simulink model "gm_uz_mpc_cost_and_optim_state_machine"  (R2021a)
settings: Solver=FixedStepAuto  StartTime=0.0  StopTime=10000*t_ADC  RelTol=1e-3
undefined symbols (not defined in the file or in its folder): A, f, IB, id_ref, iq_ref, ix_ref, iy_ref, lambda_d, lambda_q, lambda_u, lambda_x, lambda_y, Ld_over_LB, Lq_over_LB, n_rpm, omega_m, omegaB, p, psi_pm_over_psiB, Rs_over_ZB, t_ADC, t_clock, Ts_times_ZB_over_Ld, Ts_times_ZB_over_Lq, Ts_times_ZB_over_Lx, Ts_times_ZB_over_Ly, v_dc, VB
libraries: hdlmdlgenlib x73, nesl_utility x38, fl_lib x30, ee_lib x14, simulink x10, hdlsllib x2
(part 3 of 3)

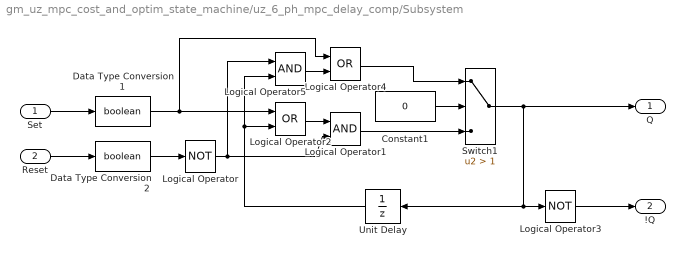
== system gm_uz_mpc_cost_and_optim_state_machine/uz_6_ph_mpc_delay_comp/Subsystem ==
  Set : Inport
  Reset : Inport  Port=2
  Constant1 : Constant  Value=0  OutDataTypeStr=uint32  SampleTime=-1
  Data Type Conversion1 : DataTypeConversion  OutDataTypeStr=boolean
  Data Type Conversion2 : DataTypeConversion  OutDataTypeStr=boolean
  Logical Operator : Logic  Operator=NOT  AllPortsSameDT=off  OutDataTypeStr=boolean
  Logical Operator1 : Logic  AllPortsSameDT=off  OutDataTypeStr=boolean
  Logical Operator2 : Logic  Operator=OR  AllPortsSameDT=off  OutDataTypeStr=boolean
  Logical Operator3 : Logic  Operator=NOT  AllPortsSameDT=off  OutDataTypeStr=boolean
  Logical Operator4 : Logic  Operator=OR  AllPortsSameDT=off  OutDataTypeStr=boolean
  Logical Operator5 : Logic  AllPortsSameDT=off  OutDataTypeStr=boolean
  Switch1 : Switch  Criteria=u2 > Threshold  Threshold=1
  Unit Delay : UnitDelay  InitialCondition=1  SampleTime=t_clock  HasFrameUpgradeWarning=on
  Q : Outport  VectorParamsAs1DForOutWhenUnconnected=off
  !Q : Outport  Port=2  VectorParamsAs1DForOutWhenUnconnected=off
  wires:
  Data Type Conversion2/1 -> Logical Operator/1
  Logical Operator1/1 -> Switch1/3
  Logical Operator5/1 -> Logical Operator4/2
  Unit Delay/1 -> Logical Operator5/2, Logical Operator2/2
  Logical Operator2/1 -> Logical Operator1/1
  Set/1 -> Data Type Conversion1/1
  Logical Operator3/1 -> !Q/1
  Switch1/1 -> Logical Operator3/1, Unit Delay/1, Q/1
  Data Type Conversion1/1 -> Logical Operator4/1, Logical Operator2/1
  Logical Operator4/1 -> Switch1/1
  Constant1/1 -> Switch1/2
  Reset/1 -> Data Type Conversion2/1
  Logical Operator/1 -> Logical Operator5/1, Logical Operator1/2

== system gm_uz_mpc_cost_and_optim_state_machine/uz_6ph_mpc_costs_and_optimization/FiniteControlSetSwitchingTable ==
  FiniteControlSetSwitchingTable : MATLAB Function  TreatAsAtomicUnit=on
  G : Outport  SampleTime=1e-08
  wires:
  FiniteControlSetSwitchingTable/1(G) -> G/1

== system gm_uz_mpc_cost_and_optim_state_machine/uz_6ph_mpc_costs_and_optimization/MATLAB Function ==
  in : Inport  OutDataTypeStr=boolean  PortDimensions=[64,12]  SampleTime=1e-08
  index : Inport  Port=2  OutDataTypeStr=uint8  PortDimensions=1  SampleTime=1e-08
  last_optim_index : Inport  Port=3  OutDataTypeStr=uint32  PortDimensions=1  SampleTime=1e-08
  MATLAB Function : MATLAB Function  TreatAsAtomicUnit=on
  G_next : Outport  SampleTime=1e-08  VectorParamsAs1DForOutWhenUnconnected=off
  G_prev : Outport  Port=2  SampleTime=1e-08
  wires:
  in/1 -> MATLAB Function/1(in)
  index/1 -> MATLAB Function/2(index)
  last_optim_index/1 -> MATLAB Function/3(last_optim_index)
  MATLAB Function/1(G_next) -> G_next/1
  MATLAB Function/2(G_prev) -> G_prev/1

== system gm_uz_mpc_cost_and_optim_state_machine/uz_6ph_mpc_costs_and_optimization/iterativesearch ==
  index : Inport  OutDataTypeStr=uint8  PortDimensions=1  SampleTime=1e-08
  cost : Inport  Port=2  OutDataTypeStr=fixdt(0, 27, 24)  PortDimensions=1  SampleTime=1e-08
  iterativesearch : MATLAB Function  TreatAsAtomicUnit=on
  iterativesearch_term1 : Terminator
  opt_idx : Outport  SampleTime=1e-08  VectorParamsAs1DForOutWhenUnconnected=off
  wires:
  index/1 -> iterativesearch/1(index)
  cost/1 -> iterativesearch/2(cost)
  iterativesearch/1(opt_idx) -> opt_idx/1
  iterativesearch/2(min_costs) -> iterativesearch_term1/1

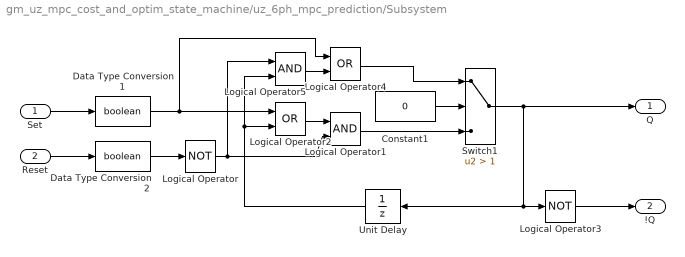
== system gm_uz_mpc_cost_and_optim_state_machine/uz_6ph_mpc_prediction/Subsystem ==
  Set : Inport
  Reset : Inport  Port=2
  Constant1 : Constant  Value=0  OutDataTypeStr=uint32  SampleTime=-1
  Data Type Conversion1 : DataTypeConversion  OutDataTypeStr=boolean
  Data Type Conversion2 : DataTypeConversion  OutDataTypeStr=boolean
  Logical Operator : Logic  Operator=NOT  AllPortsSameDT=off  OutDataTypeStr=boolean
  Logical Operator1 : Logic  AllPortsSameDT=off  OutDataTypeStr=boolean
  Logical Operator2 : Logic  Operator=OR  AllPortsSameDT=off  OutDataTypeStr=boolean
  Logical Operator3 : Logic  Operator=NOT  AllPortsSameDT=off  OutDataTypeStr=boolean
  Logical Operator4 : Logic  Operator=OR  AllPortsSameDT=off  OutDataTypeStr=boolean
  Logical Operator5 : Logic  AllPortsSameDT=off  OutDataTypeStr=boolean
  Switch1 : Switch  Criteria=u2 > Threshold  Threshold=1
  Unit Delay : UnitDelay  SampleTime=t_clock  HasFrameUpgradeWarning=on
  Q : Outport  VectorParamsAs1DForOutWhenUnconnected=off
  !Q : Outport  Port=2  VectorParamsAs1DForOutWhenUnconnected=off
  wires:
  Data Type Conversion2/1 -> Logical Operator/1
  Logical Operator1/1 -> Switch1/3
  Logical Operator5/1 -> Logical Operator4/2
  Unit Delay/1 -> Logical Operator5/2, Logical Operator2/2
  Logical Operator2/1 -> Logical Operator1/1
  Set/1 -> Data Type Conversion1/1
  Logical Operator3/1 -> !Q/1
  Switch1/1 -> Logical Operator3/1, Unit Delay/1, Q/1
  Data Type Conversion1/1 -> Logical Operator4/1, Logical Operator2/1
  Logical Operator4/1 -> Switch1/1
  Constant1/1 -> Switch1/2
  Reset/1 -> Data Type Conversion2/1
  Logical Operator/1 -> Logical Operator5/1, Logical Operator1/2

== system gm_uz_mpc_cost_and_optim_state_machine/uz_6ph_mpc_pu_voltages_vsd/Subsystem ==
  Set : Inport
  Reset : Inport  Port=2
  Constant1 : Constant  Value=0  OutDataTypeStr=uint32  SampleTime=-1
  Data Type Conversion1 : DataTypeConversion  OutDataTypeStr=boolean
  Data Type Conversion2 : DataTypeConversion  OutDataTypeStr=boolean
  Logical Operator : Logic  Operator=NOT  AllPortsSameDT=off  OutDataTypeStr=boolean
  Logical Operator1 : Logic  AllPortsSameDT=off  OutDataTypeStr=boolean
  Logical Operator2 : Logic  Operator=OR  AllPortsSameDT=off  OutDataTypeStr=boolean
  Logical Operator3 : Logic  Operator=NOT  AllPortsSameDT=off  OutDataTypeStr=boolean
  Logical Operator4 : Logic  Operator=OR  AllPortsSameDT=off  OutDataTypeStr=boolean
  Logical Operator5 : Logic  AllPortsSameDT=off  OutDataTypeStr=boolean
  Switch1 : Switch  Criteria=u2 > Threshold  Threshold=1
  Unit Delay : UnitDelay  SampleTime=t_clock  HasFrameUpgradeWarning=on
  Q : Outport  VectorParamsAs1DForOutWhenUnconnected=off
  !Q : Outport  Port=2  VectorParamsAs1DForOutWhenUnconnected=off
  wires:
  Data Type Conversion2/1 -> Logical Operator/1
  Logical Operator1/1 -> Switch1/3
  Logical Operator5/1 -> Logical Operator4/2
  Unit Delay/1 -> Logical Operator5/2, Logical Operator2/2
  Logical Operator2/1 -> Logical Operator1/1
  Set/1 -> Data Type Conversion1/1
  Logical Operator3/1 -> !Q/1
  Switch1/1 -> Logical Operator3/1, Unit Delay/1, Q/1
  Data Type Conversion1/1 -> Logical Operator4/1, Logical Operator2/1
  Logical Operator4/1 -> Switch1/1
  Constant1/1 -> Switch1/2
  Reset/1 -> Data Type Conversion2/1
  Logical Operator/1 -> Logical Operator5/1, Logical Operator1/2

== matlab function gm_uz_mpc_cost_and_optim_state_machine/uz_6ph_mpc_pu_voltages_vsd/finite_control_set ==
  settings: fimath=fimath('RoundingMethod', 'Floor','OverflowAction', 'Wrap','ProductMode', 'FullPrecision', 'SumMode', 'FullPrecision')
  data: v_DC_pu input; sin_angle input; pu_ud output; pu_uq output; pu_ux output; pu_uy output; cos_angle input; index input
function [pu_ud,pu_uq,pu_ux,pu_uy] = voltage_space_vectors(v_DC_pu, sin_angle, cos_angle, index)

fm = fimath();
v_DC_pu = fi(v_DC_pu,1,18,15,fm);
sin_angle = fi(sin_angle,1,18,16,fm);
cos_angle = fi(cos_angle,1,18,16,fm);

% u_d-voltages lookup factors alpha/beta
vd_pu = fi([0.000000,  0.000000;
0.333333,  -0.000000;
-0.166667,  0.288675;
0.166667,  0.288675;
-0.166667,  -0.288675;
0.166667,  -0.288675;
-0.333333,  0.000000;
0.000000,  0.000000;
0.288675,  0.166667;
0.622008,  0.166667;
0.122008,  0.455342;
0.455342,  0.455342;
0.122008,  -0.122008;
0.455342,  -0.122008;
-0.044658,  0.166667;
0.288675,  0.166667;
-0.288675,  0.166667;
0.044658,  0.166667;
-0.455342,  0.455342;
-0.122008,  0.455342;
-0.455342,  -0.122008;
-0.122008,  -0.122008;
-0.622008,  0.166667;
-0.288675,  0.166667;
0.000000,  0.333333;
0.333333,  0.333333;
-0.166667,  0.622008;
0.166667,  0.622008;
-0.166667,  0.044658;
0.166667,  0.044658;
-0.333333,  0.333333;
0.000000,  0.333333;
-0.000000,  -0.333333;
0.333333,  -0.333333;
-0.166667,  -0.044658;
0.166667,  -0.044658;
-0.166667,  -0.622008;
0.166667,  -0.622008;
-0.333333,  -0.333333;
-0.000000,  -0.333333;
0.288675,  -0.166667;
0.622008,  -0.166667;
0.122008,  0.122008;
0.455342,  0.122008;
0.122008,  -0.455342;
0.455342,  -0.455342;
-0.044658,  -0.166667;
0.288675,  -0.166667;
-0.288675,  -0.166667;
0.044658,  -0.166667;
-0.455342,  0.122008;
-0.122008,  0.122008;
-0.455342,  -0.455342;
-0.122008,  -0.455342;
-0.622008,  -0.166667;
-0.288675,  -0.166667;
0.000000,  0.000000;
0.333333,  -0.000000;
-0.166667,  0.288675;
0.166667,  0.288675;
-0.166667,  -0.288675;
0.166667,  -0.288675;
-0.333333,  0.000000;
0.000000,  0.000000],1,18,15);

% u_q-voltages lookup factors alpha/beta
vq_pu = fi([0.000000, 0.000000;
0.333333, -0.000000;
-0.166667, 0.288675;
0.166667, 0.288675;
-0.166667, -0.288675;
0.166667, -0.288675;
-0.333333, 0.000000;
0.000000, 0.000000;
0.288675, 0.166667;
0.622008, 0.166667;
0.122008, 0.455342;
0.455342, 0.455342;
0.122008, -0.122008;
0.455342, -0.122008;
-0.044658, 0.166667;
0.288675, 0.166667;
-0.288675, 0.166667;
0.044658, 0.166667;
-0.455342, 0.455342;
-0.122008, 0.455342;
-0.455342, -0.122008;
-0.122008, -0.122008;
-0.622008, 0.166667;
-0.288675, 0.166667;
0.000000, 0.333333;
0.333333, 0.333333;
-0.166667, 0.622008;
0.166667, 0.622008;
-0.166667, 0.044658;
0.166667, 0.044658;
-0.333333, 0.333333;
0.000000, 0.333333;
-0.000000, -0.333333;
0.333333, -0.333333;
-0.166667, -0.044658;
0.166667, -0.044658;
-0.166667, -0.622008;
0.166667, -0.622008;
-0.333333, -0.333333;
-0.000000, -0.333333;
0.288675, -0.166667;
0.622008, -0.166667;
0.122008, 0.122008;
0.455342, 0.122008;
0.122008, -0.455342;
0.455342, -0.455342;
-0.044658, -0.166667;
0.288675, -0.166667;
-0.288675, -0.166667;
0.044658, -0.166667;
-0.455342, 0.122008;
-0.122008, 0.122008;
-0.455342, -0.455342;
-0.122008, -0.455342;
-0.622008, -0.166667;
-0.288675, -0.166667;
0.000000, 0.000000;
0.333333, -0.000000;
-0.166667, 0.288675;
0.166667, 0.288675;
-0.166667, -0.288675;
0.166667, -0.288675;
-0.333333, 0.000000;
0.000000, 0.000000],1,18,15);
     
% u_x-voltages
vx_pu = fi([0.000000;
0.333333;
-0.166667;
0.166667;
-0.166667;
0.166667;
-0.333333;
0.000000;
-0.288675;
0.044658;
-0.455342;
-0.122008;
-0.455342;
-0.122008;
-0.622008;
-0.288675;
0.288675;
0.622008;
0.122008;
0.455342;
0.122008;
0.455342;
-0.044658;
0.288675;
0.000000;
0.333333;
-0.166667;
0.166667;
-0.166667;
0.166667;
-0.333333;
0.000000;
-0.000000;
0.333333;
-0.166667;
0.166667;
-0.166667;
0.166667;
-0.333333;
-0.000000;
-0.288675;
0.044658;
-0.455342;
-0.122008;
-0.455342;
-0.122008;
-0.622008;
-0.288675;
0.288675;
0.622008;
0.122008;
0.455342;
0.122008;
0.455342;
-0.044658;
0.288675;
0.000000;
0.333333;
-0.166667;
0.166667;
-0.166667;
0.166667;
-0.333333;
0.000000],1,18,15);

% u_y-voltages
vy_pu = fi([0.000000;
-0.000000;
-0.288675;
-0.288675;
0.288675;
0.288675;
0.000000;
0.000000;
0.166667;
0.166667;
-0.122008;
-0.122008;
0.455342;
0.455342;
0.166667;
0.166667;
0.166667;
0.166667;
-0.122008;
-0.122008;
0.455342;
0.455342;
0.166667;
0.166667;
0.333333;
0.333333;
0.044658;
0.044658;
0.622008;
0.622008;
0.333333;
0.333333;
-0.333333;
-0.333333;
-0.622008;
-0.622008;
-0.044658;
-0.044658;
-0.333333;
-0.333333;
-0.166667;
-0.166667;
-0.455342;
-0.455342;
0.122008;
0.122008;
-0.166667;
-0.166667;
-0.166667;
-0.166667;
-0.455342;
-0.455342;
0.122008;
0.122008;
-0.166667;
-0.166667;
0.000000;
-0.000000;
-0.288675;
-0.288675;
0.288675;
0.288675;
0.000000;
0.000000],1,18,15);

pu_ud = fi(v_DC_pu * (vd_pu(index,1) * cos_angle + vd_pu(index,2) * sin_angle),1,27,24);
pu_uq = fi(v_DC_pu * (vq_pu(index,1) * -sin_angle + vq_pu(index,2) * cos_angle),1,27,24);
pu_ux = fi(v_DC_pu * vx_pu(index),1,27,24);
pu_uy = fi(v_DC_pu * vy_pu(index),1,27,24);

== matlab function gm_uz_mpc_cost_and_optim_state_machine/uz_vsd_6ph_30deg/VSD_6ph_30deg ==
  settings: fimath=fimath('RoundingMethod', 'Floor','OverflowAction', 'Wrap','ProductMode', 'FullPrecision', 'SumMode', 'FullPrecision')
  data: a1 input; alpha output; b1 input; c1 input; a2 input; b2 input; c2 input; beta output; x1 output; y1 output; z1 output; z2 output
function [alpha,beta,x1,y1,z1,z2] = fcn(a1,b1,c1,a2,b2,c2)


A = [fi(0,1,18,11) fi(0,1,18,11) fi(0,1,18,11) fi(0,1,18,11) fi(0,1,18,11) fi(0,1,18,11)]';

A =    2/6*[1    -0.5        -0.5        sqrt(3)/2   -sqrt(3)/2  0 ;
           0    sqrt(3)/2   -sqrt(3)/2  0.5         0.5         -1;
           1    -0.5        -0.5        -sqrt(3)/2  sqrt(3)/2   0 ;
           0    -sqrt(3)/2  sqrt(3)/2   0.5         0.5         -1;
           0.5   0.5          0.5          0           0           0 ;
           0    0           0           0.5          0.5          0.5] * [a1 b1 c1 a2 b2 c2]';

alpha = fi(A(1),1,18,11);
beta = fi(A(2),1,18,11);
x1 = fi(A(3),1,18,11);
y1 = fi(A(4),1,18,11);
z1 = fi(A(5),1,18,11);
z2 = fi(A(6),1,18,11);

== matlab function gm_uz_mpc_cost_and_optim_state_machine/uz_6ph_mpc_costs_and_optimization/MATLAB Function/MATLAB Function ==
  settings: fimath=fimath('RoundingMethod', 'Floor','OverflowAction', 'Wrap','ProductMode', 'FullPrecision', 'SumMode', 'FullPrecision')
  data: in input; G_next output; index input; last_optim_index input; G_prev output
function [G_next,G_prev] = get_switch_positions(in,index,last_optim_index)
%#codegen
G_next = in(index,[1 3 5 7 9 11]);
G_prev = in(last_optim_index,[1 3 5 7 9 11]);

== matlab function gm_uz_mpc_cost_and_optim_state_machine/uz_6ph_mpc_costs_and_optimization/iterativesearch/iterativesearch ==
  data: index input; opt_idx output; cost input; min_costs output
function [opt_idx,min_costs] = fcn(index, cost)
%#codegen

persistent cost_old
if isempty(cost_old)
    cost_old = fi(4.98,0,27,24);
end

persistent index_old
if isempty(index_old)
    index_old = uint8(1);
end

persistent opt_idx_old
if isempty(opt_idx_old)
    opt_idx_old = uint8(1);
end


if (index < 63)       
       
if (index ~= index_old)
   if (cost <= cost_old)
       opt_idx_old = index; 
       cost_old = cost;
   else
    
    
   end
   index_old = index;
end

else
       cost_old = fi(4.98,0,27,24);
end

min_costs = cost_old;
opt_idx = opt_idx_old;

== matlab function gm_uz_mpc_cost_and_optim_state_machine/uz_6ph_mpc_costs_and_optimization/FiniteControlSetSwitchingTable/FiniteControlSetSwitchingTable ==
  settings: fimath=fimath('RoundingMethod', 'Floor','OverflowAction', 'Wrap','ProductMode', 'FullPrecision', 'SumMode', 'FullPrecision')
  data: G output
function G  = switchingTable

% -------------------------------------------------------------------
%  Generated by MATLAB on 14-Oct-2020 14:52:37
%  MATLAB version: 9.4.0.813654 (R2018a)
% -------------------------------------------------------------------
                                         

s1_v = boolean([0; 1; 0; 1; 0; 1; 0; 1; 0; 1; 0; 1; 0; 1; 0; 1; 0; 1; 0; 1; 0; ...
        1; 0; 1; 0; 1; 0; 1; 0; 1; 0; 1; 0; 1; 0; 1; 0; 1; 0; 1; 0; 1; ...
        0; 1; 0; 1; 0; 1; 0; 1; 0; 1; 0; 1; 0; 1; 0; 1; 0; 1; 0; 1; 0; ...
        1]);


s2_v = boolean([1; 0; 1; 0; 1; 0; 1; 0; 1; 0; 1; 0; 1; 0; 1; 0; 1; 0; 1; 0; 1; ...
        0; 1; 0; 1; 0; 1; 0; 1; 0; 1; 0; 1; 0; 1; 0; 1; 0; 1; 0; 1; 0; ...
        1; 0; 1; 0; 1; 0; 1; 0; 1; 0; 1; 0; 1; 0; 1; 0; 1; 0; 1; 0; 1; ...
        0]);


s3_v = boolean([0; 0; 1; 1; 0; 0; 1; 1; 0; 0; 1; 1; 0; 0; 1; 1; 0; 0; 1; 1; 0; ...
        0; 1; 1; 0; 0; 1; 1; 0; 0; 1; 1; 0; 0; 1; 1; 0; 0; 1; 1; 0; 0; ...
        1; 1; 0; 0; 1; 1; 0; 0; 1; 1; 0; 0; 1; 1; 0; 0; 1; 1; 0; 0; 1; ...
        1]);


s4_v = boolean([1; 1; 0; 0; 1; 1; 0; 0; 1; 1; 0; 0; 1; 1; 0; 0; 1; 1; 0; 0; 1; ...
        1; 0; 0; 1; 1; 0; 0; 1; 1; 0; 0; 1; 1; 0; 0; 1; 1; 0; 0; 1; 1; ...
        0; 0; 1; 1; 0; 0; 1; 1; 0; 0; 1; 1; 0; 0; 1; 1; 0; 0; 1; 1; 0; ...
        0]);


s5_v = boolean([0; 0; 0; 0; 1; 1; 1; 1; 0; 0; 0; 0; 1; 1; 1; 1; 0; 0; 0; 0; 1; ...
        1; 1; 1; 0; 0; 0; 0; 1; 1; 1; 1; 0; 0; 0; 0; 1; 1; 1; 1; 0; 0; ...
        0; 0; 1; 1; 1; 1; 0; 0; 0; 0; 1; 1; 1; 1; 0; 0; 0; 0; 1; 1; 1; ...
        1]);


s6_v = boolean([1; 1; 1; 1; 0; 0; 0; 0; 1; 1; 1; 1; 0; 0; 0; 0; 1; 1; 1; 1; 0; ...
        0; 0; 0; 1; 1; 1; 1; 0; 0; 0; 0; 1; 1; 1; 1; 0; 0; 0; 0; 1; 1; ...
        1; 1; 0; 0; 0; 0; 1; 1; 1; 1; 0; 0; 0; 0; 1; 1; 1; 1; 0; 0; 0; ...
        0]);


s7_v = boolean([0; 0; 0; 0; 0; 0; 0; 0; 1; 1; 1; 1; 1; 1; 1; 1; 0; 0; 0; 0; 0; ...
        0; 0; 0; 1; 1; 1; 1; 1; 1; 1; 1; 0; 0; 0; 0; 0; 0; 0; 0; 1; 1; ...
        1; 1; 1; 1; 1; 1; 0; 0; 0; 0; 0; 0; 0; 0; 1; 1; 1; 1; 1; 1; 1; ...
        1]);


s8_v = boolean([1; 1; 1; 1; 1; 1; 1; 1; 0; 0; 0; 0; 0; 0; 0; 0; 1; 1; 1; 1; 1; ...
        1; 1; 1; 0; 0; 0; 0; 0; 0; 0; 0; 1; 1; 1; 1; 1; 1; 1; 1; 0; 0; ...
        0; 0; 0; 0; 0; 0; 1; 1; 1; 1; 1; 1; 1; 1; 0; 0; 0; 0; 0; 0; 0; ...
        0]);


s9_v = boolean([0; 0; 0; 0; 0; 0; 0; 0; 0; 0; 0; 0; 0; 0; 0; 0; 1; 1; 1; 1; 1; ...
        1; 1; 1; 1; 1; 1; 1; 1; 1; 1; 1; 0; 0; 0; 0; 0; 0; 0; 0; 0; 0; ...
        0; 0; 0; 0; 0; 0; 1; 1; 1; 1; 1; 1; 1; 1; 1; 1; 1; 1; 1; 1; 1; ...
        1]);


s10_v = boolean([1; 1; 1; 1; 1; 1; 1; 1; 1; 1; 1; 1; 1; 1; 1; 1; 0; 0; 0; 0; 0; ...
         0; 0; 0; 0; 0; 0; 0; 0; 0; 0; 0; 1; 1; 1; 1; 1; 1; 1; 1; 1; 1; ...
         1; 1; 1; 1; 1; 1; 0; 0; 0; 0; 0; 0; 0; 0; 0; 0; 0; 0; 0; 0; 0; ...
         0]);


s11_v = boolean([0; 0; 0; 0; 0; 0; 0; 0; 0; 0; 0; 0; 0; 0; 0; 0; 0; 0; 0; 0; 0; ...
         0; 0; 0; 0; 0; 0; 0; 0; 0; 0; 0; 1; 1; 1; 1; 1; 1; 1; 1; 1; 1; ...
         1; 1; 1; 1; 1; 1; 1; 1; 1; 1; 1; 1; 1; 1; 1; 1; 1; 1; 1; 1; 1; ...
         1]);


s12_v = boolean([1; 1; 1; 1; 1; 1; 1; 1; 1; 1; 1; 1; 1; 1; 1; 1; 1; 1; 1; 1; 1; ...
         1; 1; 1; 1; 1; 1; 1; 1; 1; 1; 1; 0; 0; 0; 0; 0; 0; 0; 0; 0; 0; ...
         0; 0; 0; 0; 0; 0; 0; 0; 0; 0; 0; 0; 0; 0; 0; 0; 0; 0; 0; 0; 0; ...
         0]);
     
G = [s1_v, s2_v, s3_v, s4_v, s5_v, s6_v, s7_v, s8_v, s9_v, s10_v, s11_v, s12_v];
